simulink model "turtleCtrlFollower"  (R2017a)
settings: Solver=FixedStepAuto  StartTime=0.0  StopTime=inf  FixedStep=0.1  RelTol=1e-3
undefined symbols (not defined in the file or in its folder): Angular, Linear, magnitude
libraries: robotlib x11, simulink x9, TurtleCtrlLib x4, simulink_extras x1
settings Model: Creator=igeorgie  LastModifiedBy=igeorgie
settings SolverCC: AutoInsertRateTranBlk=on

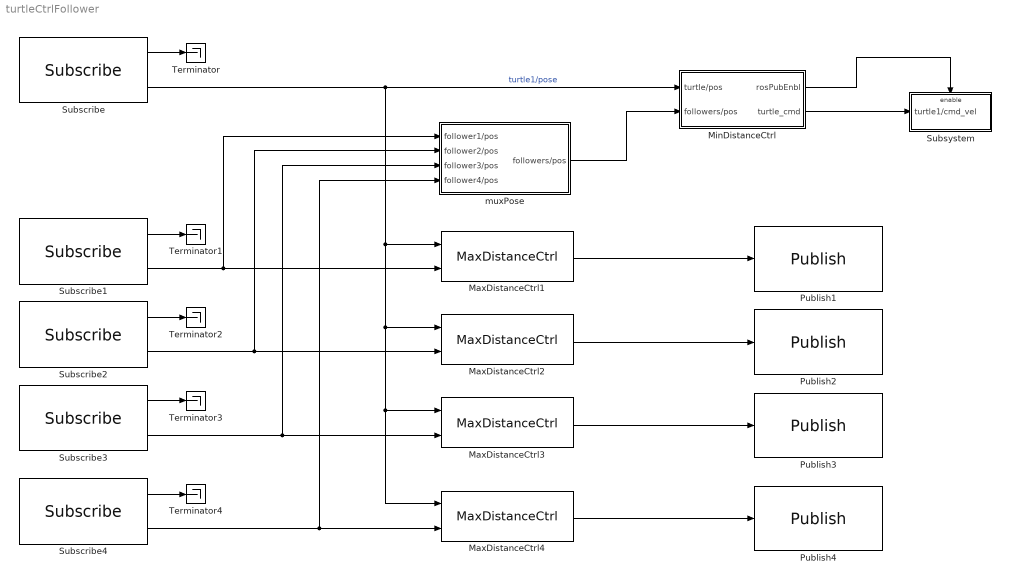
== system turtleCtrlFollower ==
  MaxDistanceCtrl1 : TurtleCtrlLib/MaxDistanceCtrl  p_gain_linear=4  p_gain_angular=3  max_distance=2.5
  MaxDistanceCtrl2 : TurtleCtrlLib/MaxDistanceCtrl  p_gain_linear=1  p_gain_angular=10  max_distance=1
  MaxDistanceCtrl3 : TurtleCtrlLib/MaxDistanceCtrl  p_gain_linear=5  p_gain_angular=1  max_distance=2.2
  MaxDistanceCtrl4 : TurtleCtrlLib/MaxDistanceCtrl  p_gain_linear=6  p_gain_angular=1  max_distance=0.5
  MinDistanceCtrl : Subsystem
  Publish1 : robotlib/Publish  SourceLibraryInfo=This block requires Robotics System Toolbox  topicSource=Select from ROS network  topic=/follower1/cmd_vel  messageType=geometry_msgs/Twist  messageQueueLength=1
      settings: SourceProductBaseCode=RO
  Publish2 : robotlib/Publish  SourceLibraryInfo=This block requires Robotics System Toolbox  topicSource=Select from ROS network  topic=/follower2/cmd_vel  messageType=geometry_msgs/Twist  messageQueueLength=1
      settings: SourceProductBaseCode=RO
  Publish3 : robotlib/Publish  SourceLibraryInfo=This block requires Robotics System Toolbox  topicSource=Select from ROS network  topic=/follower3/cmd_vel  messageType=geometry_msgs/Twist  messageQueueLength=1
      settings: SourceProductBaseCode=RO
  Publish4 : robotlib/Publish  SourceLibraryInfo=This block requires Robotics System Toolbox  topicSource=Select from ROS network  topic=/follower4/cmd_vel  messageType=geometry_msgs/Twist  messageQueueLength=1
      settings: SourceProductBaseCode=RO
  Subscribe : robotlib/Subscribe  SourceLibraryInfo=This block requires Robotics System Toolbox  topicSource=Select from ROS network  topic=/turtle1/pose  messageType=turtlesim/Pose  sampleTime=-1  messageQueueLength=1
      settings: SourceProductBaseCode=RO
  Subscribe1 : robotlib/Subscribe  SourceLibraryInfo=This block requires Robotics System Toolbox  topicSource=Select from ROS network  topic=/follower1/pose  messageType=turtlesim/Pose  sampleTime=-1  messageQueueLength=1
      settings: SourceProductBaseCode=RO
  Subscribe2 : robotlib/Subscribe  SourceLibraryInfo=This block requires Robotics System Toolbox  topicSource=Select from ROS network  topic=/follower2/pose  messageType=turtlesim/Pose  sampleTime=-1  messageQueueLength=1
      settings: SourceProductBaseCode=RO
  Subscribe3 : robotlib/Subscribe  SourceLibraryInfo=This block requires Robotics System Toolbox  topicSource=Select from ROS network  topic=/follower3/pose  messageType=turtlesim/Pose  sampleTime=-1  messageQueueLength=1
      settings: SourceProductBaseCode=RO
  Subscribe4 : robotlib/Subscribe  SourceLibraryInfo=This block requires Robotics System Toolbox  topicSource=Select from ROS network  topic=/follower4/pose  messageType=turtlesim/Pose  sampleTime=-1  messageQueueLength=1
      settings: SourceProductBaseCode=RO
  Subsystem : Subsystem
  Terminator{,1..4} (5 alike) : Terminator
  muxPose : Subsystem  TreatAsAtomicUnit=on
  wires:
  Subscribe/1 -> Terminator/1
  Subscribe/2 -> MaxDistanceCtrl4/1, MaxDistanceCtrl3/1, MaxDistanceCtrl2/1, MaxDistanceCtrl1/1, MinDistanceCtrl/1(turtle/pos)  "turtle1/pose"
  Subscribe1/1 -> Terminator1/1
  Subscribe2/1 -> Terminator2/1
  Subscribe1/2 -> MaxDistanceCtrl1/2, muxPose/1(follower1/pos)
  Subscribe2/2 -> MaxDistanceCtrl2/2, muxPose/2(follower2/pos)
  MaxDistanceCtrl1/1 -> Publish1/1
  MaxDistanceCtrl2/1 -> Publish2/1
  MinDistanceCtrl/2(turtle_cmd) -> Subsystem/1(turtle1/cmd_vel)
  MinDistanceCtrl/1(rosPubEnbl) -> Subsystem/Enable
  muxPose/1(followers/pos) -> MinDistanceCtrl/2(followers/pos)
  Subscribe3/1 -> Terminator3/1
  Subscribe3/2 -> muxPose/3(follower3/pos), MaxDistanceCtrl3/2
  Subscribe4/2 -> muxPose/4(follower4/pos), MaxDistanceCtrl4/2
  Subscribe4/1 -> Terminator4/1
  MaxDistanceCtrl3/1 -> Publish3/1
  MaxDistanceCtrl4/1 -> Publish4/1

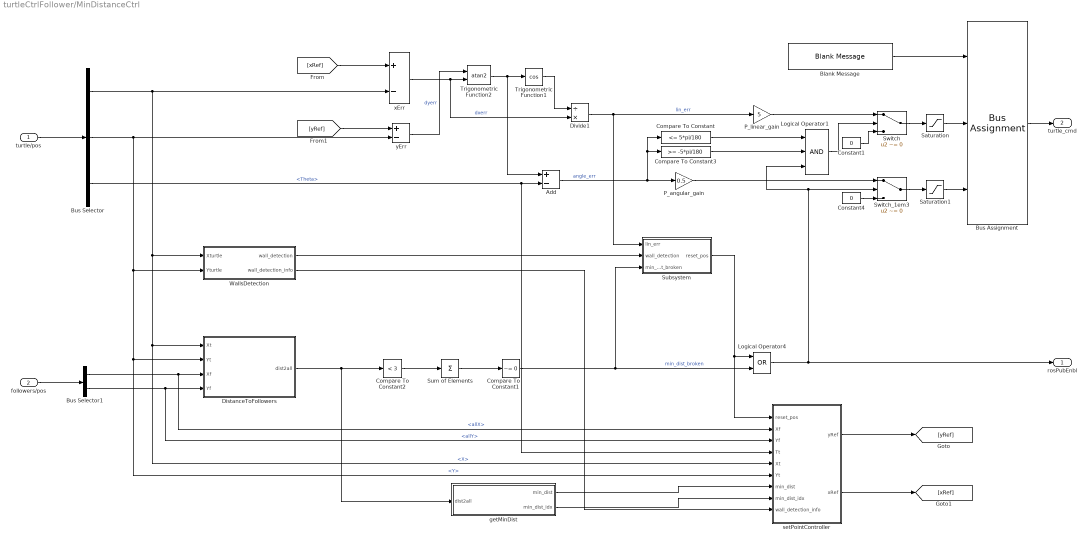
== system turtleCtrlFollower/MinDistanceCtrl ==
  turtle/pos : Inport
  followers/pos : Inport  Port=2
  Add : Sum  Inputs=+-
  Blank Message : robotlib/Blank Message  SourceLibraryInfo=This block requires Robotics System Toolbox  messageType=geometry_msgs/Twist  SampleTime=inf
      settings: SourceProductBaseCode=RO
  Bus Assignment : BusAssignment  AssignedSignals=Linear.X,Angular.Z
  Bus Selector : BusSelector  OutputSignals=X,Y,Theta
  Bus Selector1 : BusSelector  OutputSignals=allX,allY
  Compare To Constant : simulink/Logic and Bit Operations/Compare To Constant  relop=<=  const=5*pi/180  OutDataTypeStr=boolean
  Compare To Constant1 : simulink/Logic and Bit Operations/Compare To Constant  relop=~=  const=0  OutDataTypeStr=boolean
  Compare To Constant2 : simulink/Logic and Bit Operations/Compare To Constant  relop=<  const=3  OutDataTypeStr=boolean
  Compare To Constant3 : simulink/Logic and Bit Operations/Compare To Constant  relop=>=  const=-5*pi/180  OutDataTypeStr=boolean
  Constant1 : Constant  Value=0
  Constant4 : Constant  Value=0
  DistanceToFollowers : Subsystem  TreatAsAtomicUnit=on
  Divide1 : Product  Inputs=/*
  Logical Operator1 : Logic  Inputs=3  AllPortsSameDT=off  OutDataTypeStr=boolean
  Logical Operator4 : Logic  Operator=OR  AllPortsSameDT=off  OutDataTypeStr=boolean
  P_angular_gain : Gain  Gain=0.5
  P_linear_gain : Gain  Gain=5
  Saturation : Saturate  UpperLimit=1  LowerLimit=-1
  Saturation1 : Saturate  UpperLimit=10  LowerLimit=-10
  Subsystem : Subsystem
  Sum of Elements : Sum  Inputs=+
  Switch : Switch  Criteria=u2 ~= 0
  Switch_1em3 : Switch  Criteria=u2 ~= 0  Threshold=1e-3
  Trigonometric Function1 : Trigonometry  Operator=cos
  Trigonometric Function2 : Trigonometry  Operator=atan2
  WallsDetection : Subsystem  TreatAsAtomicUnit=on
  getMinDist : Subsystem
  setPointController : Subsystem
  xErr : Sum  Inputs=+-
  yErr : Sum  Inputs=+-
  rosPubEnbl : Outport
  turtle_cmd : Outport  Port=2
  wires:
  Switch/1 -> Saturation/1
  yErr/1 -> Trigonometric Function2/1  "dyerr"
  xErr/1 -> Divide1/2, Trigonometric Function2/2  "dxerr"
  Divide1/1 -> Subsystem/1(lin_err), P_linear_gain/1  "lin_err"
  Trigonometric Function1/1 -> Divide1/1
  Trigonometric Function2/1 -> Trigonometric Function1/1, Add/1
  turtle/pos/1 -> Bus Selector/1
  Blank Message/1 -> Bus Assignment/1
  Bus Assignment/1 -> turtle_cmd/1
  Bus Selector/1 -> xErr/2, setPointController/5(Xt), DistanceToFollowers/1(Xt), WallsDetection/1(Xturtle)  "<X>"
  Bus Selector/3 -> setPointController/4(Tt), Add/2  "<Theta>"
  Switch_1em3/1 -> Saturation1/1
  Sum of Elements/1 -> Compare To Constant1/1
  DistanceToFollowers/1(dist2all) -> getMinDist/1(dist2all), Compare To Constant2/1
  Compare To Constant2/1 -> Sum of Elements/1
  P_linear_gain/1 -> Switch/1
  Compare To Constant/1 -> Logical Operator1/1
  Compare To Constant3/1 -> Logical Operator1/2
  Add/1 -> P_angular_gain/1, Compare To Constant/1, Compare To Constant3/1  "angle_err"
  Logical Operator1/1 -> Switch/2
  Constant1/1 -> Switch/3
  Constant4/1 -> Switch_1em3/3
  followers/pos/1 -> Bus Selector1/1
  Bus Selector1/1 -> setPointController/2(Xf), DistanceToFollowers/3(Xf)  "<allX>"
  Bus Selector1/2 -> setPointController/3(Yf), DistanceToFollowers/4(Yf)  "<allY>"
  setPointController/1(yRef) -> [yRef]
  setPointController/2(xRef) -> [xRef]
  Saturation/1 -> Bus Assignment/2
  Saturation1/1 -> Bus Assignment/3
  Bus Selector/2 -> DistanceToFollowers/2(Yt), setPointController/6(Yt), WallsDetection/2(Yturtle), yErr/2  "<Y>"
  Compare To Constant1/1 -> Subsystem/3(min_dist_broken), Logical Operator4/2  "min_dist_broken"
  [xRef] -> xErr/1
  [yRef] -> yErr/1
  getMinDist/1(min_dist) -> setPointController/7(min_dist)
  getMinDist/2(min_dist_idx) -> setPointController/8(min_dist_idx)
  Logical Operator4/1 -> Logical Operator1/3, Switch_1em3/2, rosPubEnbl/1
  Subsystem/1(reset_pos) -> setPointController/1(reset_pos), Logical Operator4/1
  WallsDetection/1(wall_detection) -> Subsystem/2(wall_detection)
  P_angular_gain/1 -> Switch_1em3/1
  WallsDetection/2(wall_detection_info) -> setPointController/9(wall_detection_info)

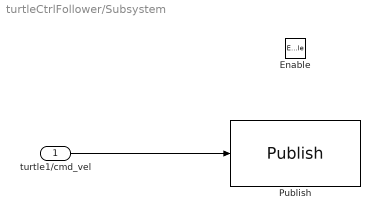
== system turtleCtrlFollower/Subsystem ==
  turtle1/cmd_vel : Inport
  Enable : EnablePort
  Publish : robotlib/Publish  SourceLibraryInfo=This block requires Robotics System Toolbox  topicSource=Select from ROS network  topic=/turtle1/cmd_vel  messageType=geometry_msgs/Twist  messageQueueLength=1
      settings: SourceProductBaseCode=RO
  wires:
  turtle1/cmd_vel/1 -> Publish/1

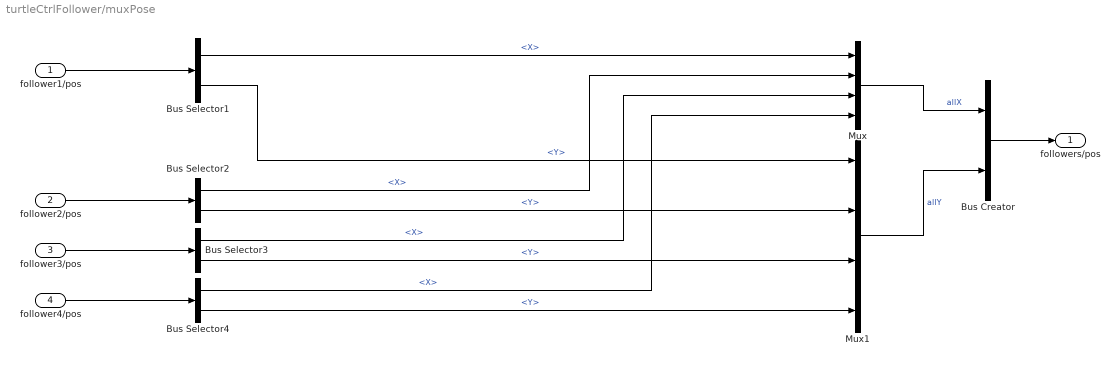
== system turtleCtrlFollower/muxPose ==
  follower1/pos : Inport
  follower2/pos : Inport  Port=2
  follower3/pos : Inport  Port=3
  follower4/pos : Inport  Port=4
  Bus Creator : BusCreator  Inputs=2
  Bus Selector{1..4} (4 alike) : BusSelector  OutputSignals=X,Y
  Mux : Mux
  Mux1 : Mux
  followers/pos : Outport
  wires:
  Bus Selector1/2 -> Mux1/1  "<Y>"
  Bus Selector1/1 -> Mux/1  "<X>"
  follower2/pos/1 -> Bus Selector2/1
  follower1/pos/1 -> Bus Selector1/1
  Mux/1 -> Bus Creator/1  "allX"
  Mux1/1 -> Bus Creator/2  "allY"
  Bus Selector2/1 -> Mux/2  "<X>"
  Bus Selector2/2 -> Mux1/2  "<Y>"
  Bus Creator/1 -> followers/pos/1
  follower3/pos/1 -> Bus Selector3/1
  follower4/pos/1 -> Bus Selector4/1
  Bus Selector3/1 -> Mux/3  "<X>"
  Bus Selector4/1 -> Mux/4  "<X>"
  Bus Selector3/2 -> Mux1/3  "<Y>"
  Bus Selector4/2 -> Mux1/4  "<Y>"

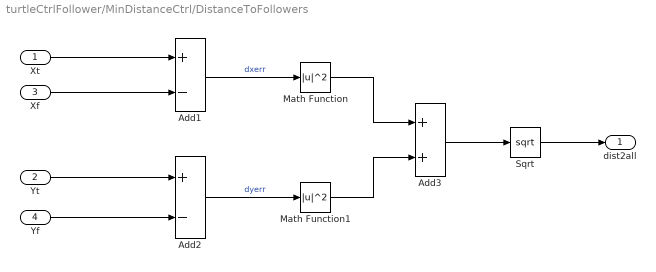
== system turtleCtrlFollower/MinDistanceCtrl/DistanceToFollowers ==
  Xt : Inport
  Yt : Inport  Port=2
  Xf : Inport  Port=3
  Yf : Inport  Port=4
  Add1 : Sum  Inputs=+-
  Add2 : Sum  Inputs=+-
  Add3 : Sum
  Math Function : Math  Operator=magnitude^2  SaturateOnIntegerOverflow=on
  Math Function1 : Math  Operator=magnitude^2  SaturateOnIntegerOverflow=on
  Sqrt : Sqrt  SaturateOnIntegerOverflow=on
  dist2all : Outport
  wires:
  Yt/1 -> Add2/1
  Xf/1 -> Add1/2
  Math Function1/1 -> Add3/2
  Add2/1 -> Math Function1/1  "dyerr"
  Add3/1 -> Sqrt/1
  Yf/1 -> Add2/2
  Sqrt/1 -> dist2all/1
  Xt/1 -> Add1/1
  Add1/1 -> Math Function/1  "dxerr"
  Math Function/1 -> Add3/1

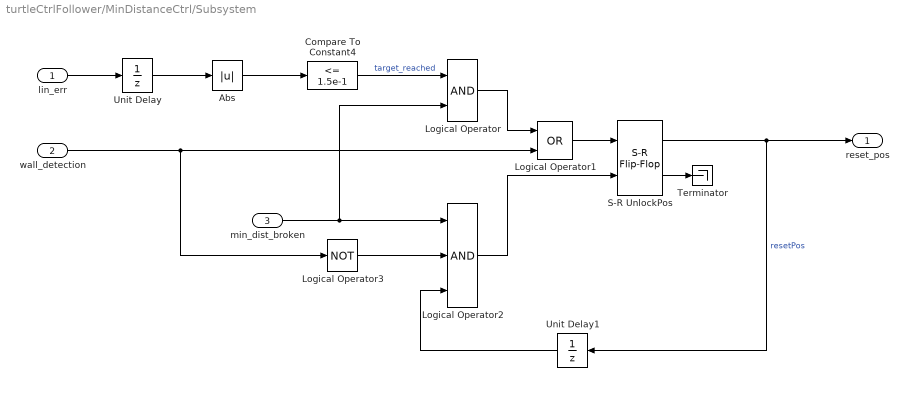
== system turtleCtrlFollower/MinDistanceCtrl/Subsystem ==
  lin_err : Inport
  wall_detection : Inport  Port=2
  min_dist_broken : Inport  Port=3
  Abs : Abs
  Compare To Constant4 : simulink/Logic and Bit Operations/Compare To Constant  relop=<=  const=1.5e-1  OutDataTypeStr=boolean
  Logical Operator : Logic  AllPortsSameDT=off  OutDataTypeStr=boolean
  Logical Operator1 : Logic  Operator=OR  AllPortsSameDT=off  OutDataTypeStr=boolean
  Logical Operator2 : Logic  Inputs=3  AllPortsSameDT=off  OutDataTypeStr=boolean
  Logical Operator3 : Logic  Operator=NOT  AllPortsSameDT=off  OutDataTypeStr=boolean
  S-R UnlockPos : simulink_extras/Flip Flops/S-R Flip-Flop  initial_condition=0
  Terminator : Terminator
  Unit Delay : UnitDelay  InitialCondition=11  SampleTime=-1
  Unit Delay1 : UnitDelay  InitialCondition=11  SampleTime=-1
  reset_pos : Outport
  wires:
  lin_err/1 -> Unit Delay/1
  min_dist_broken/1 -> Logical Operator2/1, Logical Operator/2
  Abs/1 -> Compare To Constant4/1
  Logical Operator2/1 -> S-R UnlockPos/2
  Unit Delay/1 -> Abs/1
  Unit Delay1/1 -> Logical Operator2/3
  Compare To Constant4/1 -> Logical Operator/1  "target_reached"
  Logical Operator/1 -> Logical Operator1/1
  wall_detection/1 -> Logical Operator1/2, Logical Operator3/1
  S-R UnlockPos/2 -> Terminator/1
  S-R UnlockPos/1 -> Unit Delay1/1, reset_pos/1  "resetPos"
  Logical Operator3/1 -> Logical Operator2/2
  Logical Operator1/1 -> S-R UnlockPos/1

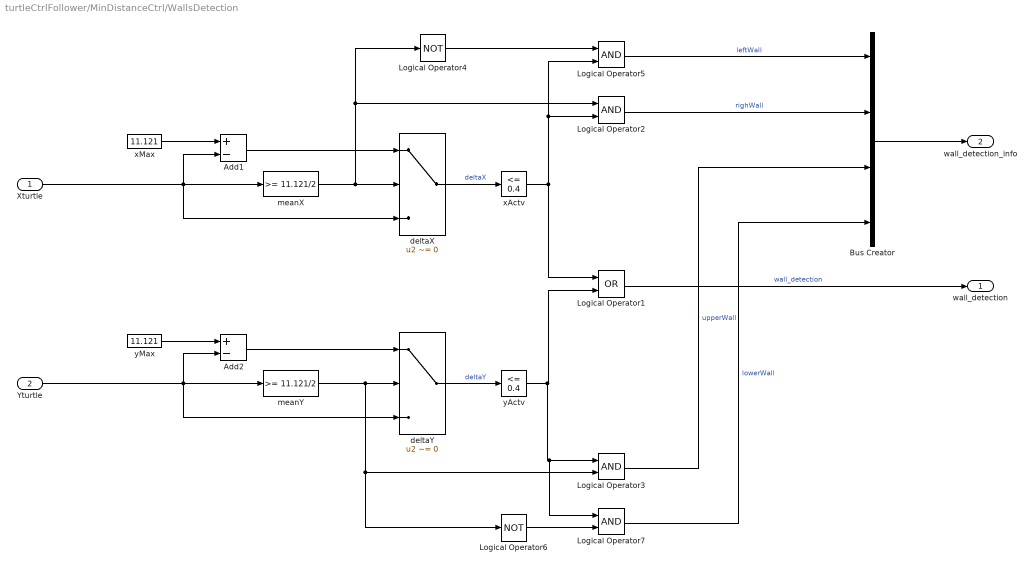
== system turtleCtrlFollower/MinDistanceCtrl/WallsDetection ==
  Xturtle : Inport
  Yturtle : Inport  Port=2
  Add1 : Sum  Inputs=+-
  Add2 : Sum  Inputs=+-
  Bus Creator : BusCreator  Inputs=4
  Logical Operator1 : Logic  Operator=OR  AllPortsSameDT=off  OutDataTypeStr=boolean
  Logical Operator{2..3,5,7} (4 alike) : Logic  AllPortsSameDT=off  OutDataTypeStr=boolean
  Logical Operator4 : Logic  Operator=NOT  AllPortsSameDT=off  OutDataTypeStr=boolean
  Logical Operator6 : Logic  Operator=NOT  AllPortsSameDT=off  OutDataTypeStr=boolean
  deltaX : Switch  Criteria=u2 ~= 0  Threshold=5.5
  deltaY : Switch  Criteria=u2 ~= 0  Threshold=5.5
  meanX : simulink/Logic and Bit Operations/Compare To Constant  relop=>=  const=11.121/2  OutDataTypeStr=boolean
  meanY : simulink/Logic and Bit Operations/Compare To Constant  relop=>=  const=11.121/2  OutDataTypeStr=boolean
  xActv : simulink/Logic and Bit Operations/Compare To Constant  relop=<=  const=0.4  OutDataTypeStr=boolean
  xMax : Constant  Value=11.121
  yActv : simulink/Logic and Bit Operations/Compare To Constant  relop=<=  const=0.4  OutDataTypeStr=boolean
  yMax : Constant  Value=11.121
  wall_detection : Outport
  wall_detection_info : Outport  Port=2
  wires:
  Xturtle/1 -> meanX/1, deltaX/3, Add1/2
  deltaX/1 -> xActv/1  "deltaX"
  Add1/1 -> deltaX/1
  xMax/1 -> Add1/1
  meanX/1 -> Logical Operator4/1, Logical Operator2/1, deltaX/2
  xActv/1 -> Logical Operator1/1, Logical Operator5/2, Logical Operator2/2
  yMax/1 -> Add2/1
  Add2/1 -> deltaY/1
  Yturtle/1 -> Add2/2, deltaY/3, meanY/1
  deltaY/1 -> yActv/1  "deltaY"
  yActv/1 -> Logical Operator1/2, Logical Operator7/1, Logical Operator3/1
  Logical Operator1/1 -> wall_detection/1  "wall_detection"
  meanY/1 -> Logical Operator3/2, Logical Operator6/1, deltaY/2
  Logical Operator3/1 -> Bus Creator/3  "upperWall"
  Logical Operator2/1 -> Bus Creator/2  "righWall"
  Logical Operator4/1 -> Logical Operator5/1
  Logical Operator5/1 -> Bus Creator/1  "leftWall"
  Logical Operator6/1 -> Logical Operator7/2
  Logical Operator7/1 -> Bus Creator/4  "lowerWall"
  Bus Creator/1 -> wall_detection_info/1

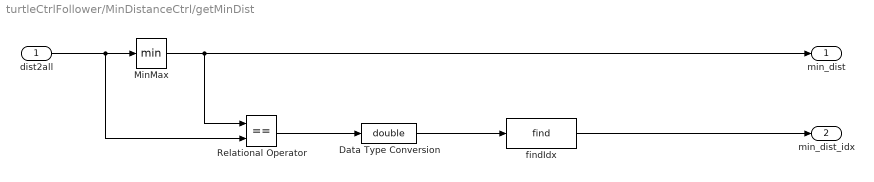
== system turtleCtrlFollower/MinDistanceCtrl/getMinDist ==
  dist2all : Inport
  Data Type Conversion : DataTypeConversion  OutDataTypeStr=double
  MinMax : MinMax
  Relational Operator : RelationalOperator  Operator===  OutDataTypeStr=boolean  RndMeth=Simplest
  findIdx : MATLABFcn  MATLABFcn=find
  min_dist : Outport
  min_dist_idx : Outport  Port=2
  wires:
  dist2all/1 -> Relational Operator/2, MinMax/1
  MinMax/1 -> min_dist/1, Relational Operator/1
  Relational Operator/1 -> Data Type Conversion/1
  Data Type Conversion/1 -> findIdx/1
  findIdx/1 -> min_dist_idx/1

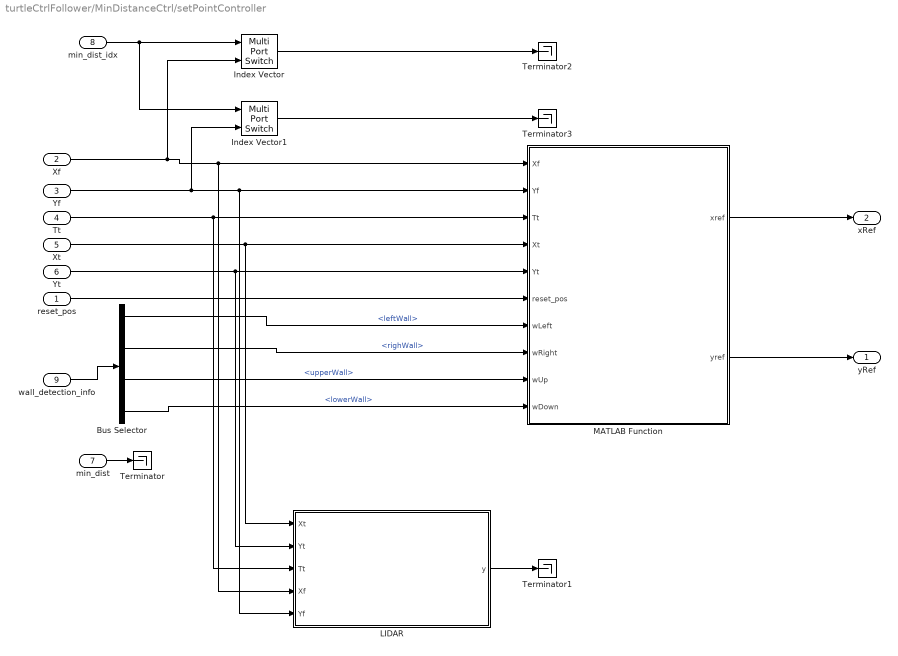
== system turtleCtrlFollower/MinDistanceCtrl/setPointController ==
  reset_pos : Inport
  Xf : Inport  Port=2
  Yf : Inport  Port=3
  Tt : Inport  Port=4
  Xt : Inport  Port=5
  Yt : Inport  Port=6
  min_dist : Inport  Port=7
  min_dist_idx : Inport  Port=8
  wall_detection_info : Inport  Port=9
  Bus Selector : BusSelector  OutputSignals=leftWall,righWall,upperWall,lowerWall
  Index Vector : MultiPortSwitch  Inputs=1
  Index Vector1 : MultiPortSwitch  Inputs=1
  LIDAR : MATLAB Function  TreatAsAtomicUnit=on
  MATLAB Function : MATLAB Function  TreatAsAtomicUnit=on
  Terminator{,1..3} (4 alike) : Terminator
  yRef : Outport
  xRef : Outport  Port=2
  wires:
  Yf/1 -> Index Vector1/2, LIDAR/5(Yf), MATLAB Function/2(Yf)
  Xf/1 -> LIDAR/4(Xf), MATLAB Function/1(Xf), Index Vector/2
  MATLAB Function/1(xref) -> xRef/1
  MATLAB Function/2(yref) -> yRef/1
  Xt/1 -> LIDAR/1(Xt), MATLAB Function/4(Xt)
  Yt/1 -> LIDAR/2(Yt), MATLAB Function/5(Yt)
  reset_pos/1 -> MATLAB Function/6(reset_pos)
  Index Vector/1 -> Terminator2/1
  Index Vector1/1 -> Terminator3/1
  min_dist_idx/1 -> Index Vector/1, Index Vector1/1
  min_dist/1 -> Terminator/1
  wall_detection_info/1 -> Bus Selector/1
  Bus Selector/1 -> MATLAB Function/7(wLeft)  "<leftWall>"
  Bus Selector/2 -> MATLAB Function/8(wRight)  "<righWall>"
  Bus Selector/3 -> MATLAB Function/9(wUp)  "<upperWall>"
  Bus Selector/4 -> MATLAB Function/10(wDown)  "<lowerWall>"
  Tt/1 -> LIDAR/3(Tt), MATLAB Function/3(Tt)
  LIDAR/1(y) -> Terminator1/1

== matlab function turtleCtrlFollower/MinDistanceCtrl/setPointController/LIDAR ==
  data: Xt input; Yt input; Tt input; Xf input; y output; Yf input

function y = lidarFcn(Xt,Yt,Tt,Xf,Yf)
y=0;

figure(1); clf; hold on;
lidarAngle=pi/2;
lidarPoints=30;
lidarRange = 4;

followerRadius = 0.3
Ymax = single(11.0);
Xmax = single(11.0);

if(Tt < 0)
    turtleTheta = 2*pi + Tt;
else
    turtleTheta = Tt;
end;

loAngle = turtleTheta - lidarAngle/2;
hiAngle = turtleTheta + lidarAngle/2;

lidarScanAngles = linspace(loAngle,hiAngle,lidarPoints)';
tmpIdx = find(lidarScanAngles < 0);
lidarScanAngles(tmpIdx) = 2*pi + lidarScanAngles(tmpIdx);

bias = Yt - Xt.*tan(lidarScanAngles);
slope = tan(lidarScanAngles);
rays = [slope bias];

xLidar = Xt + (lidarRange).*cos(lidarScanAngles);
yLidar = Yt + (lidarRange).*sin(lidarScanAngles);

tmpX=single(0);
tmpY=single(0);
rayIdx=1;
epi=pi/20000;
for rayIdx=1:length(rays)
    if ((lidarScanAngles(rayIdx) > -epi) && (lidarScanAngles(rayIdx) < epi))
        tmpX = Xmax;
        tmpY = Yt;
    elseif (lidarScanAngles(rayIdx) > (pi/2) -epi) && (lidarScanAngles(rayIdx) < (pi/2) + epi)
        tmpX = Xt;
        tmpY = Ymax;
    elseif (lidarScanAngles(rayIdx) > pi - epi) && (lidarScanAngles(rayIdx) < pi + epi)
        tmpX = single(0);
        tmpY = Yt;
    elseif (lidarScanAngles(rayIdx) > (3*pi/2) -epi) && (lidarScanAngles(rayIdx) < (3*pi/2) + epi)
        tmpX = Xt;
        tmpY = single(0);
    else
        if(lidarScanAngles(rayIdx) > 0 && lidarScanAngles(rayIdx) < pi)
            tmpX = (Ymax-rays(rayIdx,2))/rays(rayIdx,1);
            tmpY = Ymax;
        end
        
        if(lidarScanAngles(rayIdx) > pi && lidarScanAngles(rayIdx) < 2*pi)
            tmpX = -rays(rayIdx,2)/rays(rayIdx,1);
            tmpY = single(0);
        end
    end
    
    if tmpX < 0
        tmpX = single(0);
        tmpY = polyval(rays(rayIdx,:),tmpX);
    elseif tmpX > Xmax
        tmpX = Xmax;
        tmpY = polyval(rays(rayIdx,:),tmpX);
    else
    end
    
    tmpZ=zeros(rayIdx,1);
    tmpZ(rayIdx) = single(norm([Xt Yt]-[tmpX tmpY]));
    
    if(tmpZ(rayIdx) <= lidarRange)
        xLidar(rayIdx,1) = Xt + (tmpZ(rayIdx)).*cos(lidarScanAngles(rayIdx));
        yLidar(rayIdx,1) = Yt + (tmpZ(rayIdx)).*sin(lidarScanAngles(rayIdx));
        
        xRay = Xt:0.2:xLidar(rayIdx,1);
        yRay = polyval(rays(rayIdx,:),xRay);
        figure(1),plot(xRay,yRay,'--g');
    else
%         tmpZ(rayIdx) = nan;
%         xRay = Xt:0.2:xLidar(rayIdx,1);
%         yRay = polyval(rays(rayIdx,:),xRay);
%         figure(1),plot(xRay,yRay,'--g')
    end
end

targetAngle = atan2([Yf-Yt],[Xf-Xt]);

tIdx=find(targetAngle < 0);
targetAngle(tIdx) = 2*pi + targetAngle(tIdx);

zmin=ones(rayIdx,1)*100;
for(followerIdx=1:length(targetAngle))
    targetDiff = lidarScanAngles -targetAngle(followerIdx);
    [val,idxClosestRay] = min(abs(targetDiff));
    
    followerCenter = [Xf(followerIdx) Yf(followerIdx)];
    followerCircle = [followerCenter followerRadius];
    
    for rayIdx=1:lidarPoints
        [xcross,ycross] = linecirc_(rays(rayIdx,1),rays(rayIdx,2),followerCircle(1),followerCircle(2),followerCircle(3));
%         [xcross,ycross] = linecirc_(-1.1034,11.6138,2.0671,9.3705,0.9000);
        
        intersect = 0;
        dist1 = nan;
        dist2 = nan;
        if(~isnan(xcross(1)))
            dist1 = double(norm([Xt Yt] - [xcross(1) ycross(1)]));
            intersect = intersect + 1;
        end
        
        if(~isnan(xcross(2)))
            dist2 = double(norm([Xt Yt] - [xcross(2) ycross(2)]));
            intersect = intersect + 1;
        end
        
        if intersect ~= 0
            if dist1 <= dist2
                xmin = xcross(1);
                ymin = ycross(1);
                distmin = double(dist1);
            else
                xmin = xcross(2);
                ymin = ycross(2);
                distmin = double(dist2);
            end
            
            if distmin < zmin(rayIdx)
                zmin(rayIdx) = distmin;
            end
            
            crossAngle = atan2([ymin-Yt],[xmin-Xt]);
            tmpIdx = find(crossAngle < 0);
            crossAngle(tmpIdx) = 2*pi + crossAngle(tmpIdx);
            
            if (crossAngle  > lidarScanAngles(rayIdx)-pi/2000) && (crossAngle  < lidarScanAngles(rayIdx)+pi/2000)
                if distmin < lidarRange
                    xLidar(rayIdx,1) = Xt + distmin*cos(lidarScanAngles(rayIdx));
                    yLidar(rayIdx,1) = Yt + distmin*sin(lidarScanAngles(rayIdx));
                    tmpZ(rayIdx) = distmin;
                    
                    xRay = Xt:0.2:xLidar(rayIdx,1);
                    yRay = polyval(rays(rayIdx,:),xRay);
                    figure(1),plot(xRay,yRay,'--m');
                end
            end            
        else
%                         xRay = Xt:0.2:xLidar(rayIdx,1);
%                         yRay = polyval(rays(rayIdx,:),xRay);
%                         figure(1),plot(xRay,yRay,'.c')
        end    
    end
    
    xFollower = Xf(followerIdx) + followerRadius.*cos(0:pi/100:2*pi);
    yFollower = Yf(followerIdx) + followerRadius.*sin(0:pi/100:2*pi);
    figure(1),plot(xFollower,yFollower,'.y');
end

lidarDistance = tmpZ';
%lidarOut = [lidarScanAngles,lidarDistance];

nanIdx = find(isnan(tmpZ));
valIdx = find(~isnan(tmpZ));

% coeffFree = rays(nanIdx,:);
% xRayFree = arrayfun(@(n) linspace(Xt,xLidar(n),10),(1:length(coeffFree)),'UniformOutput',false)
% yRayFree = arrayfun(@(n)polyval(coeffFree(n,:),xRayFree{n}),(1:length(coeffFree))','UniformOutput',false);
% cellfun(@(x,y) plot(x,y),xRayFree,yRayFree')

plot(Xt,Yt,'o',xLidar(valIdx),yLidar(valIdx),'*m',xLidar(nanIdx),yLidar(nanIdx),'.g',Xf,Yf,'+y');
axis([0 11 0 11]);
hold off
end

function [x,y]=linecirc_(slope,intercpt,centerx,centery,radius) 
  
if nargin ~= 5;  error('Incorrect number of arguments');  end 
 
%  Input consistency test 
 
if ~isequal(size(slope),size(intercpt),size(centerx),size(centery),size(radius),[1,1]) 
	     error('Inputs must be scalars') 
elseif ~isreal([slope intercpt centerx centery radius]) 
		error('inputs must be real') 
elseif radius<=0 
		error('radius must be positive') 
end 
 
 
% find the cases of infinite slope and handle them separately 
if ~isinf(slope) 
	% From the law of cosines 
 
	a=1+slope.^2; 
	b=2*(slope.*(intercpt-centery)-centerx); 
	c=centery.^2+centerx.^2+intercpt.^2-2*centery.*intercpt-radius.^2; 
    x=[NaN NaN];
    xtmp = roots([a,b,c])'; 
 
	%  Make NaN's if they don't intersect. 
    imag_tmp = sum(abs(imag(xtmp)));
	if imag_tmp ~= 0
		x=[NaN NaN]; y=[NaN NaN]; 
	else 
		y=double([intercpt intercpt]+[slope slope].*real(xtmp)); 
        x=double(real(xtmp));
	end 
 
% vertical slope case 
elseif abs(centerx-intercpt)>radius  % They don't intercept 
	x=[NaN;NaN]; y=[NaN;NaN]; 
else 
	x=double([intercpt intercpt]); 
	step=sqrt(radius^2-(intercpt-centerx)^2); 
	y=double(centery+[step,-step]); 
end 
end

== matlab function turtleCtrlFollower/MinDistanceCtrl/setPointController/MATLAB Function ==
  data: Xf input; xref output; Yf input; Tt input; yref output; Xt input; Yt input; reset_pos input; wLeft input; wRight input; wUp input; wDown input
function [xref,yref]= fcn(Xf,Yf,Tt,Xt,Yt,reset_pos,wLeft,wRight,wUp,wDown)

%lidarFcn(Xt,Yt,Tt,Xf,Yf,pi/2,30,3);

coeff_followers = polyfit(Xf,Yf,1);

fi=atan(coeff_followers(1));

%find ortogonal angle
if(tan(fi)>0)
    si=(pi/2) + double(fi);
elseif(tan(fi)<0)
    %for fi > 90?
    si=double(fi)-(pi/2);
else
    si=pi/2;%tbd
end

bt = Yt - Xt*tan(si);
coeff_turtle=[tan(si) bt];

if(reset_pos ==1 )
    Yf_aprox = polyval(coeff_followers,Xt);
    [xref yref] = calcUnlockPos(wLeft,wRight,wUp,wDown);
else
    Yf_aprox = polyval(coeff_followers,Xt);
    [xref yref] = calcNextPos(Yt,Yf_aprox,coeff_turtle,coeff_followers);
end
x = 0:0.1:11;
y1 = polyval(coeff_followers,x);
y2 = polyval(coeff_turtle,x);

x_cross = (bt - coeff_followers(2))/(tan(fi)-tan(si));
y_cross = polyval(coeff_followers,x_cross);

ni=0:pi/25:2*pi;
x_cycle_min = Xt+2*cos(ni);
y_cycle_min = Yt+2*sin(ni);

x_cycle_max = Xt + 4*cos(ni);
y_cycle_max = Yt + 4*sin(ni);

%plot(x,y1,x,y2,'--g',Xf(1),Yf(1),'o',Xf(2),Yf(2),'o',Xf(3),Yf(3),'o',Xf(4),Yf(4),'o',xref,yref,'r+',Xt,Yt,'^',x_cross,y_cross,'mx',x_cycle_min,y_cycle_min,'.m',x_cycle_max,y_cycle_max,'.m','MarkerSize',10,'LineWidth',3)
axis([0 11.5 0 11.5])
end

function [xref, yref] = calcNextPos(Yt,Yf_aprox,coeff_turtle,coeff_followers)
tan_si=coeff_turtle(1);
bt = coeff_turtle(2);

tan_fi = coeff_followers(1)

if(Yt > Yf_aprox && tan_fi>0)...%positive slope and +Ypos
        || (Yt > Yf_aprox && tan_fi<0)...%negative slope +Ypos
        yref = double(11.);
    xref = double((11-bt)/tan_si);%xt_ymax
    if(xref>11)
        xref = double(11);
        yref = double(polyval(coeff_turtle,xref));
    elseif(xref< 0)
        xref = double(0);
        yref = double(polyval(coeff_turtle,xref));
    end
elseif(Yt < Yf_aprox && tan_fi<0)...%negative slope and -Ypos
        || (Yt < Yf_aprox && tan_fi>0)%positive slope -Ypos
    yref=double(0.);
    xref = double((0 -bt)/tan_si);%xt_ymin
    if(xref>11)
        xref = double(11);
        yref = double(polyval(coeff_turtle,xref));
    elseif(xref< 0)
        xref = double(0);
        yref = double(polyval(coeff_turtle,xref));
    end
else
    %tbd
    xref=double(5.5);
    yref=double(5.5);
end
end

function [xref, yref] = calcUnlockPos(wLeft,wRight,wUp,wDown)
xref=double(5.5);
yref=double(5.5);

if(wLeft==1)
    xref=double(10);
end

if(wRight==1)
    xref=double(1);
end

if(wUp==1)
    yref=double(1);
end

if(wDown==1)
    yref=double(10);
end

end

% function [x,y]=linecirc(slope,intercpt,centerx,centery,radius)
% 
% %LINECIRC  Find the intersections of a circle and a line in cartesian space
% %
% %  [xout,yout] = LINECIRC(slope,intercpt,centerx,centery,radius) finds
% %  the points of intersection given a circle defined by a center and
% %  radius in x-y coordinates, and a line defined by slope and
% %  y-intercept, or a slope of "inf" and an x-intercept.  Two points
% %  are returned.  When the objects do not intersect, NaNs are returned.
% %  When the line is tangent to the circle, two identical points are
% %  returned. All inputs must be scalars
% %
% %  See also CIRCCIRC
% 
% %  Copyright 1996-2002 Systems Planning and Analysis, Inc. and The MathWorks, Inc.
% %  Written by:  E. Brown, E. Byrns
% %   $Revision: 1.9 $    $Date: 2002/03/20 21:25:45 $
% 
% 
% if nargin ~= 5;  error('Incorrect number of arguments');  end
% 
% %  Input consistency test
% 
% if ~isequal(size(slope),size(intercpt),size(centerx),size(centery),size(radius),[1,1])
%     error('Inputs must be scalars')
% elseif ~isreal([slope intercpt centerx centery radius])
%     error('inputs must be real')
% elseif radius<=0
%     error('radius must be positive')
% end
% 
% 
% % find the cases of infinite slope and handle them separately
% 
% if ~isinf(slope)
%     % From the law of cosines
%     
%     a=1+slope.^2;
%     b=2*(slope.*(intercpt-centery)-centerx);
%     c=centery.^2+centerx.^2+intercpt.^2-2*centery.*intercpt-radius.^2;
%     
%     x=roots([a,b,c])';
%     
%     %  Make NaN's if they don't intersect.
%     
%     if ~isreal(x)
%         x=[NaN NaN]; y=[NaN NaN];
%     else
%         y=[intercpt intercpt]+[slope slope].*x;
%     end
%     
%     % vertical slope case
% elseif abs(centerx-intercpt)>radius  % They don't intercept
%     x=[NaN;NaN]; y=[NaN;NaN];
% else
%     x=[intercpt intercpt];
%     step=sqrt(radius^2-(intercpt-centerx)^2);
%     y=centery+[step,-step];
% end
% end
% 
% 
% function lidarFcn(Xt,Yt,Tt,Xf,Yf,lidarAngle,lidarPoints,lidarRange)
% figure(1); clf; hold on;
% 
% followerRadius = 0.4
% Ymax = single(11.0);
% Xmax = single(11.0);
% 
% if(Tt < 0)
%     turtleTheta = pi - Tt;
% else
%     turtleTheta = Tt;
% end;
% 
% loAngle = turtleTheta - lidarAngle/2;
% hiAngle = turtleTheta + lidarAngle/2;
% 
% lidarScanAngles = linspace(loAngle,hiAngle,lidarPoints)';
% tmpIdx = find(lidarScanAngles < 0);
% lidarScanAngles(tmpIdx) = 2*pi + lidarScanAngles(tmpIdx);
% 
% bias = Yt - Xt.*tan(lidarScanAngles);
% slope = tan(lidarScanAngles);
% rays = [slope bias];
% 
% xLidar = Xt + (lidarRange).*cos(lidarScanAngles);
% yLidar = Yt + (lidarRange).*sin(lidarScanAngles);
% 
% tmpX=single(0);
% tmpY=single(0);
% rayIdx=1;
% epi=pi/20000;
% for rayIdx=1:length(rays)
%     if ((lidarScanAngles(rayIdx) > -epi) && (lidarScanAngles(rayIdx) < epi))
%         tmpX = Xmax;
%         tmpY = Yt;
%     elseif (lidarScanAngles(rayIdx) > (pi/2) -epi) && (lidarScanAngles(rayIdx) < (pi/2) + epi)
%         tmpX = Xt;
%         tmpY = Ymax;
%     elseif (lidarScanAngles(rayIdx) > pi - epi) && (lidarScanAngles(rayIdx) < pi + epi)
%         tmpX = single(0);
%         tmpY = Yt;
%     elseif (lidarScanAngles(rayIdx) > (3*pi/2) -epi) && (lidarScanAngles(rayIdx) < (3*pi/2) + epi)
%         tmpX = Xt;
%         tmpY = single(0);
%     else
%         if(lidarScanAngles(rayIdx) > 0 && lidarScanAngles(rayIdx) < pi)
%             tmpX = (Ymax-rays(rayIdx,2))/rays(rayIdx,1);
%             tmpY = Ymax;
%         end
%         
%         if(lidarScanAngles(rayIdx) > pi && lidarScanAngles(rayIdx) < 2*pi)
%             tmpX = -rays(rayIdx,2)/rays(rayIdx,1);
%             tmpY = single(0);
%         end
%     end
%     
%     if tmpX < 0
%         tmpX = single(0);
%         tmpY = polyval(rays(rayIdx,:),tmpX);
%     elseif tmpX > Xmax
%         tmpX = Xmax;
%         tmpY = polyval(rays(rayIdx,:),tmpX);
%     else
%     end
%     
%     tmpZ=zeros(rayIdx,1);
%     tmpZ(rayIdx) = single(norm([Xt Yt]-[tmpX tmpY]));
%     
%     if(tmpZ(rayIdx) <= lidarRange)
%         xLidar(rayIdx,1) = Xt + (tmpZ(rayIdx)).*cos(lidarScanAngles(rayIdx));
%         yLidar(rayIdx,1) = Yt + (tmpZ(rayIdx)).*sin(lidarScanAngles(rayIdx));
%         
%         xRay = Xt:0.2:xLidar(rayIdx,1);
%         yRay = polyval(rays(rayIdx,:),xRay);
%         figure(1),plot(xRay,yRay,'--g')
%     else
%         tmpZ(rayIdx) = nan;
%         xRay = Xt:0.2:xLidar(rayIdx,1);
%         yRay = polyval(rays(rayIdx,:),xRay);
%         figure(1),plot(xRay,yRay,'--g')
%     end
% end
% 
% targetAngle = atan2([Yf-Yt],[Xf-Xt]);
% 
% tIdx=find(targetAngle < 0);
% targetAngle(tIdx) = 2*pi + targetAngle(tIdx);
% 
% for(followerIdx=1:length(targetAngle))
%     targetDiff = lidarScanAngles -targetAngle(followerIdx);
%     [val,idxClosestRay] = min(abs(targetDiff));
%     
%     followerCenter = [Xf(followerIdx) Yf(followerIdx)]
%     followerCircle = [followerCenter followerRadius]
%     
%     for rayIdx=1:lidarPoints
%         [xcross,ycross] = linecirc(rays(rayIdx,1),rays(rayIdx,2),followerCircle(1),followerCircle(2),followerCircle(3));
%         
%         intersect = 0;
%         if(~isnan(xcross(1)))
%             dist1 = norm([Xt Yt] - [xcross(1) ycross(1)]);
%             intersect = intersect + 1;
%         end
%         
%         if(~isnan(xcross(2)))
%             dist2 = norm([Xt Yt] - [xcross(2) ycross(2)]);
%             intersect = intersect + 1;
%         end
%         
%         if intersect ~= 0
%             if dist1 <= dist2
%                 xmin = xcross(1);
%                 ymin = ycross(1);
%                 distmin = dist1;
%             else
%                 xmin = xcross(2);
%                 ymin = ycross(2);
%                 distmin = dist2;
%             end
%             crossAngle = atan2([ymin-Yt],[xmin-Xt]);
%             tmpIdx = find(crossAngle < 0);
%             crossAngle(tmpIdx) = 2*pi + crossAngle(tmpIdx);
%             
%             if (crossAngle  > lidarScanAngles(rayIdx)-pi/2000) && (crossAngle  < lidarScanAngles(rayIdx)+pi/2000)
%                 if distmin < lidarRange
%                     xLidar(rayIdx,1) = Xt + distmin*cos(lidarScanAngles(rayIdx));
%                     yLidar(rayIdx,1) = Yt + distmin*sin(lidarScanAngles(rayIdx));
%                     tmpZ(rayIdx) = distmin;
%                     
%                     xRay = Xt:0.2:xLidar(rayIdx,1);
%                     yRay = polyval(rays(rayIdx,:),xRay);
%                     figure(1),plot(xRay,yRay,'--m')
%                 end
%             end
%         else
%             %             xRay = Xt:0.2:xLidar(rayIdx,1);
%             %             yRay = polyval(rays(rayIdx,:),xRay);
%             %             figure(1),plot(xRay,yRay,'.c')
%         end
%     end
%     
%     xFollower = Xf(followerIdx) + followerRadius.*cos(0:pi/100:2*pi);
%     yFollower = Yf(followerIdx) + followerRadius.*sin(0:pi/100:2*pi);
%     figure(1),plot(xFollower,yFollower,'.g')
% end
% 
% lidarDistance = tmpZ';
% lidarOut = [lidarScanAngles,lidarDistance];
% 
% nanIdx = find(isnan(tmpZ));
% valIdx = find(~isnan(tmpZ));
% 
% % coeffFree = rays(nanIdx,:);
% % xRayFree = arrayfun(@(n) linspace(Xt,xLidar(n),10),(1:length(coeffFree)),'UniformOutput',false)
% % yRayFree = arrayfun(@(n)polyval(coeffFree(n,:),xRayFree{n}),(1:length(coeffFree))','UniformOutput',false);
% % cellfun(@(x,y) plot(x,y),xRayFree,yRayFree')
% 
% plot(Xt,Yt,'o',xLidar(valIdx),yLidar(valIdx),'.m',xLidar(nanIdx),yLidar(nanIdx),'.g',Xf,Yf,'+m');
% axis([0 11 0 11]);
% hold off
% end
